simulink model "KinDyn"  (R2019b)
settings: Solver=ode4  StartTime=0.0  StopTime=60  FixedStep=0.01  RelTol=1e-3  EnableMultiTasking=on
InitFcn:
  | clear all
  | U_Path
  | roboparam
undefined symbols (not defined in the file or in its folder): L, psicw10, psicw20, psicw30, psicw40, rho0, rho1, rhoH, th0, th1, v0, w0, xtrolley0, ytrolley0
libraries: simulink x3
settings Model: Creator=e0010448  LastModifiedBy=vladkhon
settings DataIOCC: LimitDataPoints=on  SaveFormat=StructureWithTime  ReturnWorkspaceOutputs=off
settings OptimizationCC: BlockReduction=off  BufferReuse=off  LifeSpan=inf
settings DebuggingCC: AlgebraicLoopMsg=none  UnconnectedInputMsg=none  UnconnectedOutputMsg=none  UnconnectedLineMsg=none  AllowSymbolicDim=off  SFUnexpectedBacktrackingDiag=warning  SFNoUnconditionalDefaultTransitionDiag=warning  SFExecutionAtInitializationDiag=none  ArithmeticOperatorsInVariantConditions=warning
settings HardwareCC: ProdBitPerPointer=32  ProdBitPerSizeT=32  ProdBitPerPtrDiffT=32  ProdLargestAtomicFloat=None  ProdIntDivRoundTo=Undefined  ProdEndianess=Unspecified  ProdWordSize=32  ProdHWDeviceType=32-bit Generic
settings ModelReferenceCC: PropagateSignalLabelsOutOfModel=off
settings SFSimCC: SimUseLocalCustomCode=off  CustomCodeUndefinedFunction=UseInterfaceOnly
settings RTWCC: RTWUseLocalCustomCode=off
settings CodeAppCC: StateflowObjectComments=on
settings GRTTargetCC: TargetLangStandard=C89/C90 (ANSI)  GeneratePreprocessorConditionals=Disable all
settings ConfigComp: CovMetricSettings=dw  CovHtmlReporting=on  CovSaveCumulativeToWorkspaceVar=on  CovSaveSingleToWorkspaceVar=on  CovExternalEMLEnable=off

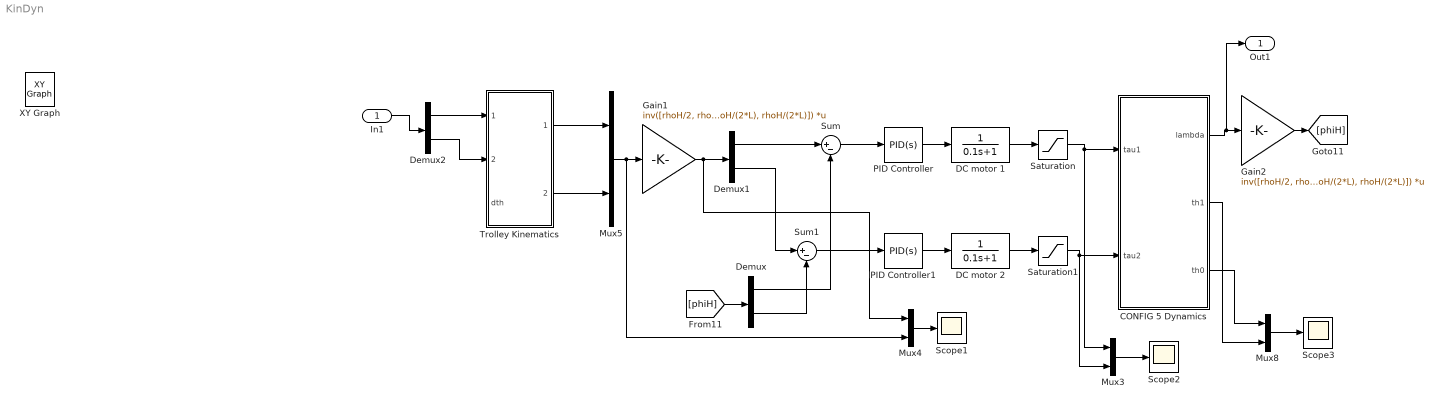
== system KinDyn ==
  In1 : Inport  PortDimensions=2  SampleTime=0  LockScale=on
  CONFIG 5 Dynamics : Subsystem
  DC motor 1 : TransferFcn  Denominator=[0.1 1]
  DC motor 2 : TransferFcn  Denominator=[0.1 1]
  Demux : Demux  Outputs=2
  Demux1 : Demux  Outputs=2
  Demux2 : Demux  Outputs=2
  Gain1 : Gain  Gain=inv([rhoH/2, rhoH/2; -rhoH/(2*L), rhoH/(2*L)])  Multiplication=Matrix(K*u)
  Gain2 : Gain  Gain=inv([rhoH/2, rhoH/2; -rhoH/(2*L), rhoH/(2*L)])  Multiplication=Matrix(K*u)
  Mux{3..5,8} (4 alike) : Mux  Inputs=2
  PID Controller : simulink/Continuous/PID Controller  Controller=PID  Form=Parallel  TimeDomain=Continuous-time  SampleTime=-1  IntegratorMethod=Forward Euler  FilterMethod=Forward Euler  ControllerParametersSource=internal  P=3  I=5  D=1  UseFilter=on  N=100  TunerSelectOption=Transfer Function Based (PID Tuner App)  InitialConditionSource=internal  InitialConditionForIntegrator=0  InitialConditionForFilter=0  DifferentiatorICPrevScaledInput=0  ExternalReset=none  TrackingMode=off  Kt=1  LimitOutput=off  UpperSaturationLimit=inf  LowerSaturationLimit=-inf  LinearizeAsGain=on  AntiWindupMode=none  Kb=1  POutMin=[]  POutMax=[]  IOutMin=[]  IOutMax=[]  DOutMin=[]  DOutMax=[]  NOutMin=[]  NOutMax=[]  SumOutMin=[]  SumOutMax=[]  SaturationOutMin=[]  SaturationOutMax=[]  PParamMin=[]  PParamMax=[]  IParamMin=[]  IParamMax=[]  DParamMin=[]  DParamMax=[]  NParamMin=[]  NParamMax=[]  KbParamMin=[]  KbParamMax=[]  KtParamMin=[]  KtParamMax=[]  KbOutMin=[]  KbOutMax=[]  KtOutMin=[]  KtOutMax=[]  IntegratorOutMin=[]  IntegratorOutMax=[]  FilterOutMin=[]  FilterOutMax=[]  SumI1OutMin=[]  SumI1OutMax=[]  SumI2OutMin=[]  SumI2OutMax=[]  SumI3OutMin=[]  SumI3OutMax=[]  SumI4OutMin=[]  SumI4OutMax=[]  SumDOutMin=[]  SumDOutMax=[]  DifferentiatorOutMin=[]  DifferentiatorOutMax=[]  FilterDiffOutCoefMin=[]  FilterDiffOutCoefMax=[]  ReciprocalOutMin=[]  ReciprocalOutMax=[]  SumDenOutMin=[]  SumDenOutMax=[]  SumNumOutMin=[]  SumNumOutMax=[]  DivideOutMin=[]  DivideOutMax=[]  IntegratorContinuousStateAttributes=''  IntegratorStateMustResolveToSignalObject=off  IntegratorRTWStateStorageClass=Auto  FilterContinuousStateAttributes=''  FilterStateMustResolveToSignalObject=off  FilterRTWStateStorageClass=Auto  ParallelPVariant=InternalParameters  IdealPVariant=Disabled  IVariant=InternalParameters  DVariant=InternalParameters  IntegratorVariant=Continuous  SatVariant=Disabled  AWVariant=Passthrough  PCopyVariant=Disabled  TRVariant=Disabled  FdbkBlocksVariant=Forward  IdealPFdbkVariant=Disabled  SatFdbkVariant=Disabled  DerivativeFilterVariant=ContFilter  NVariant=InternalParameters  NCopyVariant=Disabled  FilterICVariant=InternalICsFilter  IntegratorICVariant=InternalICs  ExternalResetVariant=Disabled  TRSumVariant=Passthrough  SumFdbkVariant=Disabled  SumVariant=Sum_PID
  PID Controller1 : simulink/Continuous/PID Controller  Controller=PID  Form=Parallel  TimeDomain=Continuous-time  SampleTime=-1  IntegratorMethod=Forward Euler  FilterMethod=Forward Euler  ControllerParametersSource=internal  P=3  I=5  D=1  UseFilter=on  N=100  TunerSelectOption=Transfer Function Based (PID Tuner App)  InitialConditionSource=internal  InitialConditionForIntegrator=0  InitialConditionForFilter=0  DifferentiatorICPrevScaledInput=0  ExternalReset=none  TrackingMode=off  Kt=1  LimitOutput=off  UpperSaturationLimit=inf  LowerSaturationLimit=-inf  LinearizeAsGain=on  AntiWindupMode=none  Kb=1  POutMin=[]  POutMax=[]  IOutMin=[]  IOutMax=[]  DOutMin=[]  DOutMax=[]  NOutMin=[]  NOutMax=[]  SumOutMin=[]  SumOutMax=[]  SaturationOutMin=[]  SaturationOutMax=[]  PParamMin=[]  PParamMax=[]  IParamMin=[]  IParamMax=[]  DParamMin=[]  DParamMax=[]  NParamMin=[]  NParamMax=[]  KbParamMin=[]  KbParamMax=[]  KtParamMin=[]  KtParamMax=[]  KbOutMin=[]  KbOutMax=[]  KtOutMin=[]  KtOutMax=[]  IntegratorOutMin=[]  IntegratorOutMax=[]  FilterOutMin=[]  FilterOutMax=[]  SumI1OutMin=[]  SumI1OutMax=[]  SumI2OutMin=[]  SumI2OutMax=[]  SumI3OutMin=[]  SumI3OutMax=[]  SumI4OutMin=[]  SumI4OutMax=[]  SumDOutMin=[]  SumDOutMax=[]  DifferentiatorOutMin=[]  DifferentiatorOutMax=[]  FilterDiffOutCoefMin=[]  FilterDiffOutCoefMax=[]  ReciprocalOutMin=[]  ReciprocalOutMax=[]  SumDenOutMin=[]  SumDenOutMax=[]  SumNumOutMin=[]  SumNumOutMax=[]  DivideOutMin=[]  DivideOutMax=[]  IntegratorContinuousStateAttributes=''  IntegratorStateMustResolveToSignalObject=off  IntegratorRTWStateStorageClass=Auto  FilterContinuousStateAttributes=''  FilterStateMustResolveToSignalObject=off  FilterRTWStateStorageClass=Auto  ParallelPVariant=InternalParameters  IdealPVariant=Disabled  IVariant=InternalParameters  DVariant=InternalParameters  IntegratorVariant=Continuous  SatVariant=Disabled  AWVariant=Passthrough  PCopyVariant=Disabled  TRVariant=Disabled  FdbkBlocksVariant=Forward  IdealPFdbkVariant=Disabled  SatFdbkVariant=Disabled  DerivativeFilterVariant=ContFilter  NVariant=InternalParameters  NCopyVariant=Disabled  FilterICVariant=InternalICsFilter  IntegratorICVariant=InternalICs  ExternalResetVariant=Disabled  TRSumVariant=Passthrough  SumFdbkVariant=Disabled  SumVariant=Sum_PID
  Saturation : Saturate  UpperLimit=40  LowerLimit=-40
  Saturation1 : Saturate  UpperLimit=40  LowerLimit=-40
  Scope1 : Scope
  Scope2 : Scope
  Scope3 : Scope
  Sum : Sum  Inputs=|+-
  Sum1 : Sum  Inputs=|+-
  Trolley Kinematics : Subsystem
  Out1 : Outport
  XY Graph : simulink/Sinks/XY Graph  IOType=viewer  xmin=-1  xmax=1  ymin=-1  ymax=1  st=-1
  wires:
  Sum/1 -> PID Controller/1
  [phiH] -> Demux/1
  Demux/1 -> Sum/2
  Demux/2 -> Sum1/2
  Sum1/1 -> PID Controller1/1
  Mux4/1 -> Scope1/1
  Mux5/1 -> Mux4/2, Gain1/1
  Gain2/1 -> [phiH]
  Demux1/1 -> Sum/1
  Demux1/2 -> Sum1/1
  Mux3/1 -> Scope2/1
  Gain1/1 -> Mux4/1, Demux1/1
  PID Controller/1 -> DC motor 1/1
  PID Controller1/1 -> DC motor 2/1
  DC motor 1/1 -> Saturation/1
  Saturation/1 -> Mux3/1, CONFIG 5 Dynamics/1(tau1)
  DC motor 2/1 -> Saturation1/1
  Saturation1/1 -> Mux3/2, CONFIG 5 Dynamics/2(tau2)
  Trolley Kinematics/1(vQcmd) -> Mux5/1
  Trolley Kinematics/2(wQcmd) -> Mux5/2
  Mux8/1 -> Scope3/1
  CONFIG 5 Dynamics/2(th1) -> Mux8/2
  CONFIG 5 Dynamics/3(th0) -> Mux8/1
  CONFIG 5 Dynamics/1(lambda) -> Out1/1, Gain2/1
  In1/1 -> Demux2/1
  Demux2/1 -> Trolley Kinematics/1(vPcmd)
  Demux2/2 -> Trolley Kinematics/2(wPcmd)

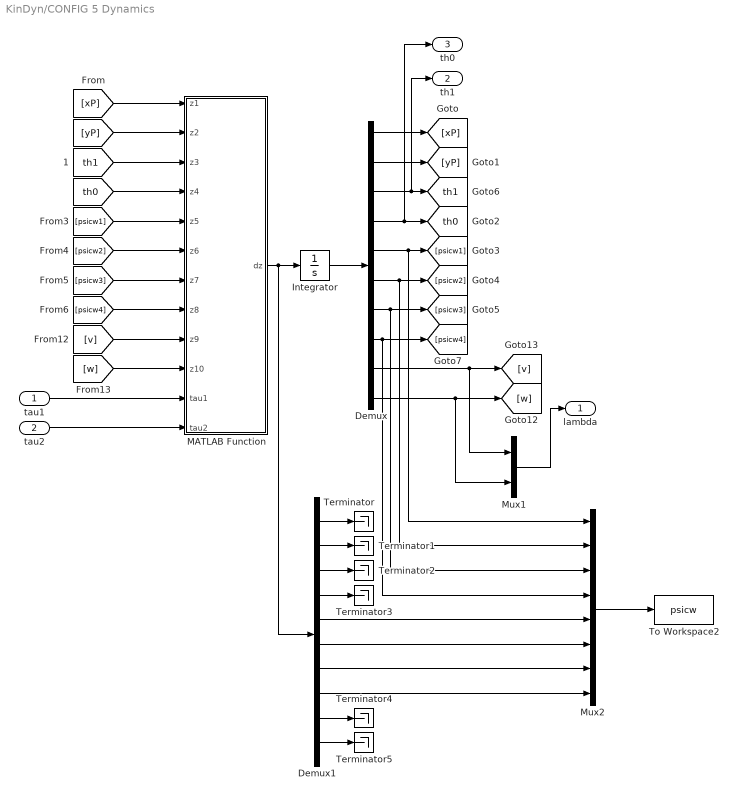
== system KinDyn/CONFIG 5 Dynamics ==
  tau1 : Inport
  tau2 : Inport  Port=2
  Demux : Demux  Outputs=10
  Demux1 : Demux  Outputs=10
  Integrator : Integrator  InitialCondition=[xtrolley0 ytrolley0 th1 th0 psicw10 psicw20 psicw30 psicw40 v0 w0]
  MATLAB Function : MATLAB Function  TreatAsAtomicUnit=on
  Mux1 : Mux  Inputs=2
  Mux2 : Mux  Inputs=8
  Terminator{,1..5} (6 alike) : Terminator
  To Workspace2 : ToWorkspace  VariableName=psicw  SaveFormat=Timeseries  SampleTime=-1
  lambda : Outport  VectorParamsAs1DForOutWhenUnconnected=off
  th1 : Outport  Port=2  VectorParamsAs1DForOutWhenUnconnected=off
  th0 : Outport  Port=3  VectorParamsAs1DForOutWhenUnconnected=off
  tag scope: th0=global, th1=global
  wires:
  Mux1/1 -> lambda/1
  Integrator/1 -> Demux/1
  Demux/10 -> Mux1/2, [w]
  Demux/9 -> Mux1/1, [v]
  Demux/8 -> [psicw4], Mux2/4
  Demux/7 -> [psicw3], Mux2/3
  Demux/6 -> [psicw2], Mux2/2
  Demux/5 -> [psicw1], Mux2/1
  Demux/2 -> [yP]
  Demux/1 -> [xP]
  MATLAB Function/1(dz) -> Demux1/1, Integrator/1
  [xP] -> MATLAB Function/1(z1)
  [yP] -> MATLAB Function/2(z2)
  [psicw1] -> MATLAB Function/5(z5)
  [psicw2] -> MATLAB Function/6(z6)
  [psicw3] -> MATLAB Function/7(z7)
  [psicw4] -> MATLAB Function/8(z8)
  [v] -> MATLAB Function/9(z9)
  [w] -> MATLAB Function/10(z10)
  [th1] -> MATLAB Function/3(z3)
  [th0] -> MATLAB Function/4(z4)
  Demux/3 -> th1/1, [th1]
  Demux/4 -> th0/1, [th0]
  tau1/1 -> MATLAB Function/11(tau1)
  tau2/1 -> MATLAB Function/12(tau2)
  Demux1/8 -> Mux2/8
  Demux1/7 -> Mux2/7
  Demux1/6 -> Mux2/6
  Demux1/5 -> Mux2/5
  Mux2/1 -> To Workspace2/1
  Demux1/1 -> Terminator/1
  Demux1/2 -> Terminator1/1
  Demux1/4 -> Terminator3/1
  Demux1/3 -> Terminator2/1
  Demux1/10 -> Terminator5/1
  Demux1/9 -> Terminator4/1

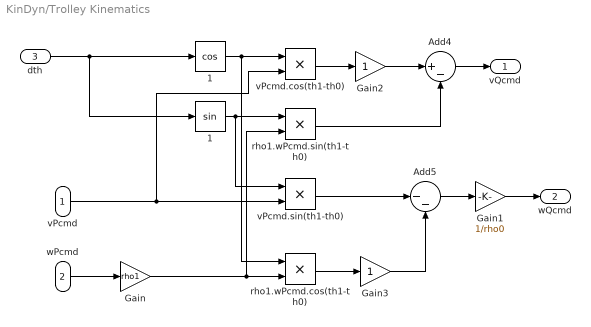
== system KinDyn/Trolley Kinematics ==
  vPcmd : Inport
  wPcmd : Inport  Port=2
  dth : Inport  Port=3
  "          1" : Trigonometry
  "         1" : Trigonometry  Operator=cos
  Add4 : Sum  Inputs=|+-
  Add5 : Sum  Inputs=|--
  Gain : Gain  Gain=rho1
  Gain1 : Gain  Gain=1/rho0
  Gain2 : Gain
  Gain3 : Gain
  rho1.wPcmd.cos(th1-th0) : Product
  rho1.wPcmd.sin(th1-th0) : Product
  vPcmd.cos(th1-th0) : Product
  vPcmd.sin(th1-th0) : Product
  vQcmd : Outport  VectorParamsAs1DForOutWhenUnconnected=off
  wQcmd : Outport  Port=2  VectorParamsAs1DForOutWhenUnconnected=off
  wires:
  "         1"/1 -> rho1.wPcmd.cos(th1-th0)/1, vPcmd.cos(th1-th0)/1
  dth/1 -> "         1"/1, "          1"/1
  "          1"/1 -> vPcmd.sin(th1-th0)/1, rho1.wPcmd.sin(th1-th0)/1
  Gain/1 -> rho1.wPcmd.sin(th1-th0)/2, rho1.wPcmd.cos(th1-th0)/2
  rho1.wPcmd.sin(th1-th0)/1 -> Add4/2
  vPcmd/1 -> vPcmd.cos(th1-th0)/2, vPcmd.sin(th1-th0)/2
  wPcmd/1 -> Gain/1
  Add5/1 -> Gain1/1
  Gain1/1 -> wQcmd/1
  vPcmd.sin(th1-th0)/1 -> Add5/1
  Add4/1 -> vQcmd/1
  vPcmd.cos(th1-th0)/1 -> Gain2/1
  Gain2/1 -> Add4/1
  rho1.wPcmd.cos(th1-th0)/1 -> Gain3/1
  Gain3/1 -> Add5/2

== matlab function KinDyn/CONFIG 5 Dynamics/MATLAB Function ==
  data: z1 input; dz output; z2 input; z3 input; z4 input; z5 input; z6 input; z7 input; z8 input; z9 input; z10 input; tau1 input; tau2 input
function dz = AXON_Dynamics_CONF5_VW_Simulink(z1,z2,z3,z4,z5,z6,z7,z8,z9,z10,tau1,tau2)
%% ODE function for the dynamics of configuration 5 that uses linear and angular velocity states
% t -> time variable
% z -> state variables  [x,y,th1,th0,psicw(4),v,w]

% variable state assignment

% position of pt P (x,y) axon orientation (th0) and trolley orientation (th1)
x = z1;
y = z2;
th1 = z3;
th0 = z4;

% caster wheel orientation (psicw_i)
psicw1 = z5;
psicw2 = z6;
psicw3 = z7;
psicw4 = z8;

% linear and angular velocity of and about point Q (v,w)
v = z9;
w = z10;

% distance in m
rho0 = 0.5;%0.5; 
rho1 = 1;%1;

L = 0.387/2;
s_l = 1.12;
s_w = 0.5;
dcw = 0.05;
dqpx = 0;  % distance bet q and P
dqcmBx = -0.648/4; % distance bet Q and Axon com
cw1x = -s_l/2;
cw1_x = cw1x;
cw3x =  s_l/2;
cw3_x = cw3x;
dpcmPx = 0;%s_l/2;

% mass in kg
mB = 50;
m_P = 15;
mH = 2;
mW = 0.7;
mCW = 1.0; 
mT = m_P + 2*mW + 2*mH + 2*mCW +mB;


% wheel radius
rhoH = 0.075;
rho_h = rhoH;
rhow = 0.06;
rho_w = rhow;
rhocw = 0.05;
rho_cw = rhocw;

e1 = (2*mH + mB)*rho1 + dpcmPx*m_P - 2*mCW*s_l; % dqpx*m_P + 2*mCW*(cw3x + cw1x) + dqcmBx*mB;
e2 = (2*mH + mB)*rho0 + dqcmBx*mB;

IWy = (1/2)*mW*rho_w^2;
IWz = (1/12)*mW*(3*rho_w^2 + 0.03^2);
ICWz = (1/12)*mCW*(3*rho_cw^2 + 0.01^2);
IPz = (1/12)*m_P*(s_l^2 + (2*s_w)^2);
IBz = (1/12)*mB*(0.3^2 + 0.6^2);
IHz = (1/12)*mH*(3*rho_h^2 + 0.03^2);
IHy = (1/2)*mH*rho_h^2;

ITw = IWz + s_w^2*mW;
ITCWz = ICWz + mCW*dcw^2;
ITB = IBz + mB*dqcmBx^2;
ITH = IHz + mH*L^2;
IT_P = IPz + m_P*dpcmPx^2;

ITz = (2*mH + mB)*rho0^2 + 2*dqcmBx*mB*rho0 + ITB + 2*ITH;
ITP = (2*mH + mB)*rho1^2 + IT_P + 2*ITw + 2*mCW*(s_w^2 + s_l^2);

T = rhoH/2*[1, 1; -1/L 1/L]; % transformation matrix for driving wheels to velocities[v;w] = T*dphiH

dphi=inv(T)*[v;w];
dphiH1 = dphi(1);   % driving wheels rotation rate (L)
dphiH2 = dphi(2);   % driving wheels rotation rate (R)


%% Config 5
%% Trolley Kinematics
% dx, dy, dth1, dth0 -> change in position and orientation
dx = cos(th1)*cos(th1-th0)*v-cos(th1)*sin(th1-th0)*rho0*w;
dy = sin(th1)*cos(th1-th0)*v-sin(th1)*sin(th1-th0)*rho0*w;
dth1 = -sin(th1-th0)/rho1*v-(cos(th1-th0)*rho0)/rho1*w;
dth0 = w;

delthd = dth1 - dth0;

%% Trolley Kinematics
% dpsicw -> caster wheel swivel rate (change in caster wheel orientation)
dpsicw1  = -(v*(2*s_w*sin(th1-th0)*sin(psicw1-th1)-s_l*sin(th1-th0)*cos(psicw1-th1)+2* ...
    cos(th1)*cos(th1-th0)*rho1*sin(psicw1)-2*sin(th1)*cos(th1-th0)*rho1*cos(psicw1))+w*rho0*(2* ...
    s_w*cos(th1-th0)*sin(psicw1-th1)-s_l*cos(th1-th0)*cos(psicw1-th1)-2*cos(th1)*sin(th1-th0)* ...
    rho1*sin(psicw1)+2*sin(th1)*sin(th1-th0)*rho1*cos(psicw1)))/(2*dcw*rho1);

dpsicw2  = (v*(2*s_w*sin(th1-th0)*sin(psicw2-th1)+s_l*sin(th1-th0)*cos(psicw2-th1)-2* ...
    cos(th1)*cos(th1-th0)*rho1*sin(psicw2)+2*sin(th1)*cos(th1-th0)*rho1*cos(psicw2))+w*rho0*(2* ...
    s_w*cos(th1-th0)*sin(psicw2-th1)+s_l*cos(th1-th0)*cos(psicw2-th1)+2*cos(th1)*sin(th1-th0) ...
    *rho1*sin(psicw2)-2*sin(th1)*sin(th1-th0)*rho1*cos(psicw2)))/(2*dcw*rho1);

dpsicw3  = -(v*(2*s_w*sin(th1-th0)*sin(psicw3-th1)+s_l*sin(th1-th0)*cos(psicw3-th1)+2* ...
    cos(th1)*cos(th1-th0)*rho1*sin(psicw3)-2*sin(th1)*cos(th1-th0)*rho1*cos(psicw3))+w*rho0*(2* ...
    s_w*cos(th1-th0)*sin(psicw3-th1)+s_l*cos(th1-th0)*cos(psicw3-th1)-2*cos(th1)*sin(th1-th0) ...
    *rho1*sin(psicw3)+2*sin(th1)*sin(th1-th0)*rho1*cos(psicw3)))/(2*dcw*rho1);

dpsicw4  = (v*(2*s_w*sin(th1-th0)*sin(psicw4-th1)-s_l*sin(th1-th0)*cos(psicw4-th1)-2* ...
    cos(th1)*cos(th1-th0)*rho1*sin(psicw4)+2*sin(th1)*cos(th1-th0)*rho1*cos(psicw4))+w*rho0*(2* ...
    s_w*cos(th1-th0)*sin(psicw4-th1)-s_l*cos(th1-th0)*cos(psicw4-th1)+2*cos(th1)*sin(th1-th0) ...
    *rho1*sin(psicw4)-2*sin(th1)*sin(th1-th0)*rho1*cos(psicw4)))/(2*dcw*rho1);

%% Dynamics: Mpp*d?/dt + npp*? + n3p*psiCW = Bpp*?
%       ? = [v;w]; ? = [?1; ?2] 

Mpp = [[(2*IHy)/rhoH^2+(ITP*sin(th1-th0)^2)/rho1^2+mT*cos(th1-th0)^2 , (ITP*cos(th1-th0)*sin(th1-th0)*rho0)/rho1^2-mT*cos(th1-th0)*sin(th1-th0)*rho0]; ...
    [(ITP*cos(th1-th0)*sin(th1-th0)*rho0)/rho1^2-mT*cos(th1-th0)*sin(th1-th0)*rho0, (2*IHy*L^2)/rhoH^2+(ITP*cos(th1-th0)^2*rho0^2)/rho1^2+mT*sin(th1-th0)^2*rho0^2-2*e2*rho0+ITz]];

npp = [[-(delthd*cos(th1-th0)*sin(th1-th0)*(mT*rho1^2-ITP))/rho1^2, -(delthd*rho0*(mT*cos(th1-th0)^2*rho1^2+ITP*sin(th1-th0)^2)+e2*(dth0)*rho1^2-e1*(dth1)*rho0*rho1)/rho1^2];...
    [(delthd*rho0*(mT*sin(th1-th0)^2*rho1^2+ITP*cos(th1-th0)^2)+e2*(dth0)*rho1^2-e1*(dth1)*rho0*rho1)/rho1^2 , (delthd*cos(th1-th0)*sin(th1-th0)*rho0^2*(mT*rho1^2-ITP))/rho1^2]];

n3p = [[(dcw*mCW*(dpsicw1)*(s_l*sin(th1-th0)*sin(psicw1-th1)+2*cos(th1-th0)*rho1*cos(psicw1-th1)+2*s_w*sin(th1-th0)*cos(psicw1-th1)))/(2*rho1) , (dcw*mCW*(dpsicw2)*(s_l*sin(th1-th0)*sin(psicw2-th1)+2*cos(th1-th0)*rho1*cos(psicw2-th1)-2*s_w*sin(th1-th0)*cos(psicw2-th1)))/(2*rho1), ...
    -(dcw*mCW*(dpsicw3)*(s_l*sin(th1-th0)*sin(psicw3-th1)-2*s_w*sin(th1-th0)*cos(psicw3-th1)-2*sin(th1)*cos(th1-th0)*rho1*sin(psicw3)-2*cos(th1)*cos(th1-th0)*rho1*cos(psicw3)))/(2*rho1) , -(dcw*mCW*(dpsicw4)*(s_l*sin(th1-th0)*sin(psicw4-th1)+2*s_w*sin(th1-th0)*cos(psicw4-th1)-2*sin(th1)*cos(th1-th0)*rho1*sin(psicw4)-2*cos(th1)*cos(th1-th0)*rho1*cos(psicw4)))/(2*rho1)];...
    [(dcw*mCW*rho0*(dpsicw1)*(s_l*cos(th1-th0)*sin(psicw1-th1)-2*sin(th1-th0)*rho1*cos(psicw1-th1)+2*s_w*cos(th1-th0)*cos(psicw1-th1)))/(2*rho1) , (dcw*mCW*rho0*(dpsicw2)*(s_l*cos(th1-th0)*sin(psicw2-th1)-2*sin(th1-th0)*rho1*cos(psicw2-th1)-2*s_w*cos(th1-th0)*cos(psicw2-th1)))/(2*rho1), ...
    -(dcw*mCW*rho0*(dpsicw3)*(s_l*cos(th1-th0)*sin(psicw3-th1)-2*s_w*cos(th1-th0)*cos(psicw3-th1)+2*sin(th1)*sin(th1-th0)*rho1*sin(psicw3)+2*cos(th1)*sin(th1-th0)*rho1*cos(psicw3)))/(2*rho1) , -(dcw*mCW*rho0*(dpsicw4)*(s_l*cos(th1-th0)*sin(psicw4-th1)+2*s_w*cos(th1-th0)*cos(psicw4-th1)+2*sin(th1)*sin(th1-th0)*rho1*sin(psicw4)+2*cos(th1)*sin(th1-th0)*rho1*cos(psicw4)))/(2*rho1)]];

Bpp = [[1/rhoH,1/rhoH];[-L/rhoH,L/rhoH]];
tau = [tau1; tau2];

% d?/dt -> equation for the solution of the linear and angular accelerations
dvw = inv(Mpp)*(Bpp*tau - npp*[v;w] - n3p*[dpsicw1;dpsicw2;dpsicw3;dpsicw4]);
dv = dvw(1);    % linear acceleration
dw = dvw(2);    % angular acceleration

dz = [dx,dy,dth1,dth0,dpsicw1, dpsicw2, dpsicw3, dpsicw4, dv, dw].';
